simulink model "MPPT_Python"  (R2022b)
settings: Solver=VariableStepAuto  StartTime=0.0  StopTime=1  RelTol=1e-3
settings Model: Creator=owner  LastModifiedBy=owner

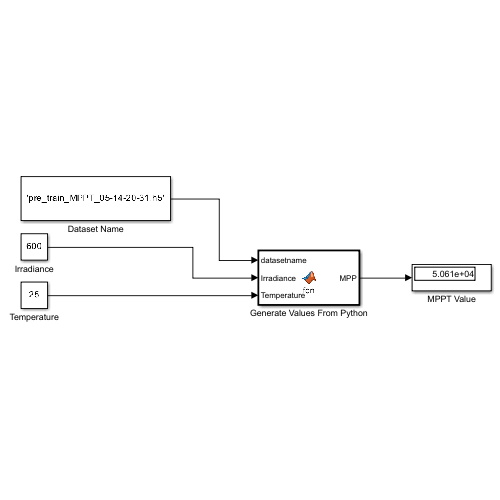
[thumbnail: Simulink's stored preview of the top-level diagram]
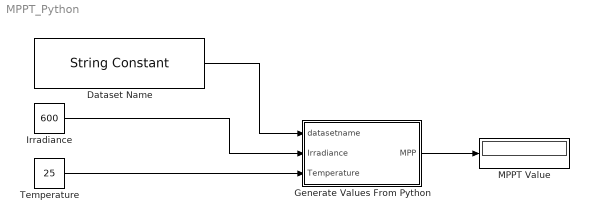
== system MPPT_Python ==
  Dataset Name : StringConstant  String='pre_train_MPPT_05-14-20-31.h5'
  Generate Values From Python : MATLAB Function  TreatAsAtomicUnit=on
  Irradiance : Constant  Value=600
  MPPT Value : Display
  Temperature : Constant  Value=25
  wires:
  Irradiance/1 -> Generate Values From Python/2(Irradiance)
  Temperature/1 -> Generate Values From Python/3(Temperature)
  Generate Values From Python/1(MPP) -> MPPT Value/1
  Dataset Name/1 -> Generate Values From Python/1(datasetname)

== matlab function MPPT_Python/Generate Values From Python ==
  data: datasetname input; MPP output; Irradiance input; Temperature input
function MPP  = fcn(datasetname, Irradiance, Temperature)
   
   % Declare py.math.cos and py.math.sin as extrinsic functions
   coder.extrinsic('py.Load_Dataset.test_MPPT');
   % Preallocate outputs
   MPP = double(0);

   MPP = py.Load_Dataset.test_MPPT(datasetname, Irradiance, Temperature);

end
